simulink model "exercise02_simulation_model_solution_partA_R2025b"  (R2025b)
settings: Solver=VariableStepAuto  StartTime=0.0  StopTime=10.0  RelTol=1e-3
PreLoadFcn:
  | exercise02_simulation_parameters
undefined symbols (not defined in the file or in its folder): g, g_vec, K_lqr_full_state, nrotor_initial_condition, nrotor_initial_conditions, nrotor_vehicle, reference, sigbuilder_block
libraries: vrlib x1
settings Model: Creator=resjoehr  LastModifiedBy=diego
settings DataIOCC: SaveFormat=Array  StreamToWks=off  ReturnWorkspaceOutputs=off

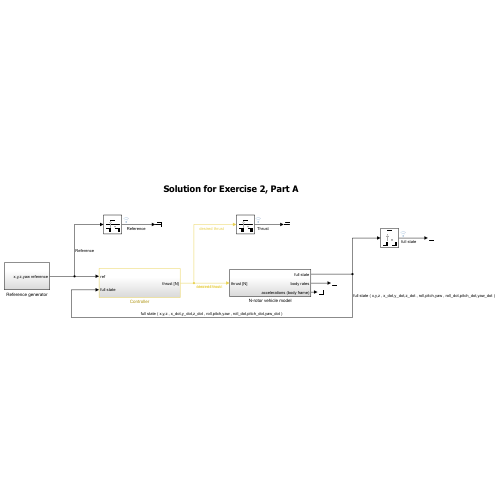
[thumbnail: Simulink's stored preview of the top-level diagram]
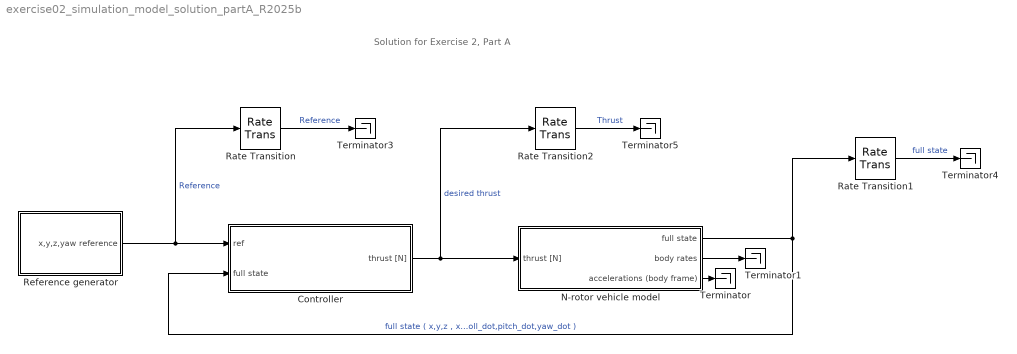
== system exercise02_simulation_model_solution_partA_R2025b ==
  note: Solution for Exercise 2, Part A
  Controller : Subsystem
  N-rotor vehicle model : Subsystem
  Rate Transition : RateTransition  OutPortSampleTime=0.05
  Rate Transition1 : RateTransition  OutPortSampleTime=0.05
  Rate Transition2 : RateTransition  OutPortSampleTime=0.05
  Reference generator : Subsystem
  Terminator{,1,3..5} (5 alike) : Terminator
  wires:
  N-rotor vehicle model/2(body rates) -> Terminator1/1
  Reference generator/1(x,y,z,yaw reference) -> Rate Transition/1, Controller/1(ref)  "Reference"
  N-rotor vehicle model/3(accelerations (body frame)) -> Terminator/1
  N-rotor vehicle model/1(full state) -> Controller/2(full state), Rate Transition1/1  "full state ( x,y,z , x_dot,y_dot,z_dot , roll,pitch,yaw , roll_dot,pitch_dot,yaw_dot )"
  Controller/1(thrust [N]) -> Rate Transition2/1, N-rotor vehicle model/1(thrust [N])  "desired thrust"
  Rate Transition1/1 -> Terminator4/1  "full state"
  Rate Transition/1 -> Terminator3/1  "Reference"
  Rate Transition2/1 -> Terminator5/1  "Thrust"

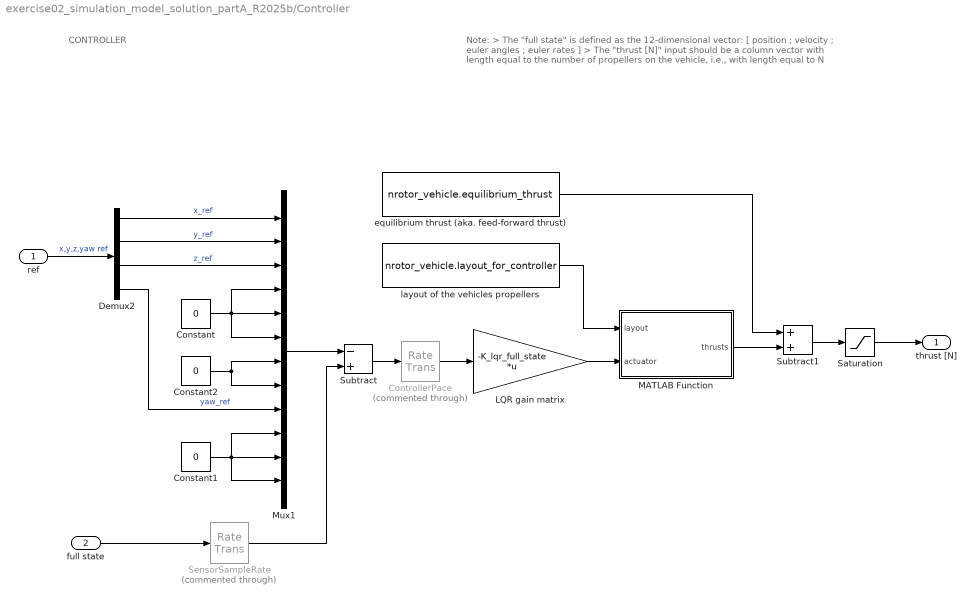
== system exercise02_simulation_model_solution_partA_R2025b/Controller ==
  note: CONTROLLER
  note: Note:
      | > The "full state" is defined as the 12-dimensional vector:
      | [ position ; velocity ; euler angles ; euler rates ]
      | > The "thrust [N]" input should be a column vector with
      | length equal to the number of propellers on the vehicle,
      | i.e., with length equal to N
  ref : Inport
  full state : Inport  Port=2
  Constant : Constant  Value=0
  Constant1 : Constant  Value=0
  Constant2 : Constant  Value=0
  ControllerPace : RateTransition  Commented=through  OutPortSampleTime=0.005
  Demux2 : Demux
  LQR gain matrix : Gain  Gain=-K_lqr_full_state  Multiplication=Matrix(K*u)
  MATLAB Function : MATLAB Function  TreatAsAtomicUnit=on
  Mux1 : Mux  Inputs=12
  Saturation : Saturate  UpperLimit=nrotor_vehicle.thrust_max  LowerLimit=nrotor_vehicle.thrust_min  ZeroCross=off
  SensorSampleRate : RateTransition  Commented=through  OutPortSampleTime=0.005
  Subtract : Sum  Inputs=-+
  Subtract1 : Sum
  equilibrium thrust (aka. feed-forward thrust) : Constant  Value=nrotor_vehicle.equilibrium_thrust
  layout of the vehicles propellers : Constant  Value=nrotor_vehicle.layout_for_controller
  thrust [N] : Outport  VectorParamsAs1DForOutWhenUnconnected=off
  wires:
  Saturation/1 -> thrust [N]/1
  ref/1 -> Demux2/1  "x,y,z,yaw ref"
  Mux1/1 -> Subtract/1
  Demux2/1 -> Mux1/1  "x_ref"
  Demux2/2 -> Mux1/2  "y_ref"
  Demux2/3 -> Mux1/3  "z_ref"
  Constant/1 -> Mux1/6, Mux1/5, Mux1/4
  full state/1 -> SensorSampleRate/1
  Subtract/1 -> ControllerPace/1
  LQR gain matrix/1 -> MATLAB Function/2(actuator)
  Subtract1/1 -> Saturation/1
  equilibrium thrust (aka. feed-forward thrust)/1 -> Subtract1/1
  Constant1/1 -> Mux1/11, Mux1/12, Mux1/10
  Constant2/1 -> Mux1/8, Mux1/7
  Demux2/4 -> Mux1/9  "yaw_ref"
  MATLAB Function/1(thrusts) -> Subtract1/2
  layout of the vehicles propellers/1 -> MATLAB Function/1(layout)
  SensorSampleRate/1 -> Subtract/2
  ControllerPace/1 -> LQR gain matrix/1

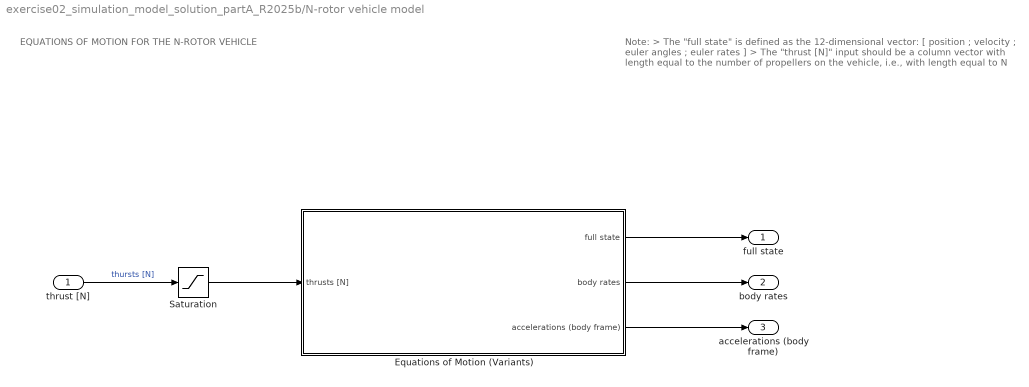
== system exercise02_simulation_model_solution_partA_R2025b/N-rotor vehicle model ==
  note: Note:
      | > The "full state" is defined as the 12-dimensional vector:
      | [ position ; velocity ; euler angles ; euler rates ]
      | > The "thrust [N]" input should be a column vector with
      | length equal to the number of propellers on the vehicle,
      | i.e., with length equal to N
  note: EQUATIONS OF MOTION FOR THE N-ROTOR VEHICLE
  thrust [N] : Inport
  Equations of Motion (Variants) : Subsystem  Variant=on  VariantControlMode=label  LabelModeActiveChoice=Choice_2
  Saturation : Saturate  UpperLimit=nrotor_vehicle.thrust_max  LowerLimit=nrotor_vehicle.thrust_min
  full state : Outport  VectorParamsAs1DForOutWhenUnconnected=off
  body rates : Outport  Port=2  VectorParamsAs1DForOutWhenUnconnected=off
  accelerations (body frame) : Outport  Port=3  VectorParamsAs1DForOutWhenUnconnected=off
  wires:
  thrust [N]/1 -> Saturation/1  "thursts [N]"
  Saturation/1 -> Equations of Motion (Variants)/1(thrusts [N])
  Equations of Motion (Variants)/2(body rates) -> body rates/1
  Equations of Motion (Variants)/1(full state) -> full state/1
  Equations of Motion (Variants)/3(accelerations (body frame)) -> accelerations (body frame)/1

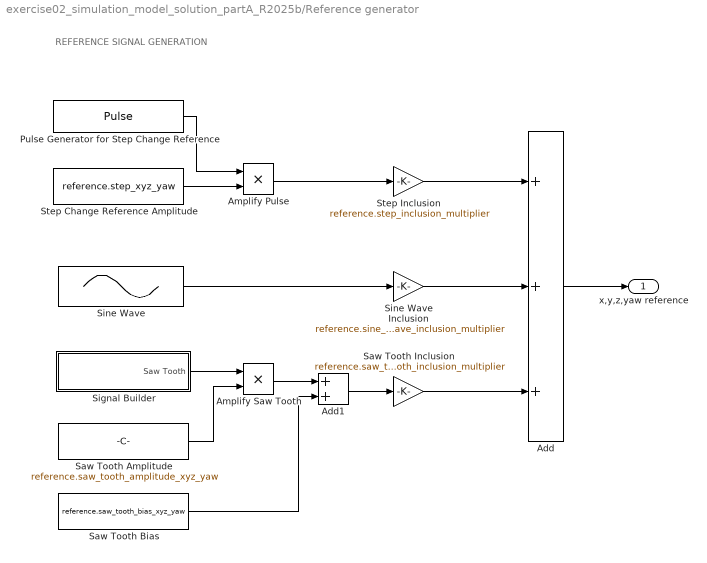
== system exercise02_simulation_model_solution_partA_R2025b/Reference generator ==
  note: REFERENCE SIGNAL GENERATION
  Add : Sum  Inputs=+++
  Add1 : Sum
  Amplify Pulse : Product
  Amplify Saw Tooth : Product
  Pulse Generator for Step Change Reference : DiscretePulseGenerator  PulseType=Time based  Period=reference.step_period*2  PulseWidth=50
  Saw Tooth Amplitude : Constant  Value=reference.saw_tooth_amplitude_xyz_yaw
  Saw Tooth Bias : Constant  Value=reference.saw_tooth_bias_xyz_yaw
  Saw Tooth Inclusion : Gain  Gain=reference.saw_tooth_inclusion_multiplier
  Signal Builder : Subsystem  Tag=STV Subsys  LoadFcn=sigbuilder_block('load');  StartFcn=sigbuilder_block('start');  StopFcn=sigbuilder_block('stop');  ClipboardFcn=sigbuilder_block('clipboard');  mask(Sigbuilder block){tuvar=[0:10]}
      mask help: Simulink:masks:SigbuilderBlock_MD
      mask init:
      | if ~strcmp(get_param(bdroot(gcbh),'SimulationStatus'),'stopped') tuvar = sigbuilder_block('maskInit'); end
      settings: CopyFcn=sigbuilder_block('copy');  DeleteFcn=sigbuilder_block('delete');  ModelCloseFcn=sigbuilder_block('modelClose');  PreSaveFcn=sigbuilder_block('preSave');  PauseFcn=sigbuilder_block('pause');  ContinueFcn=sigbuilder_block('continue');  NameChangeFcn=sigbuilder_block('namechange');  OpenFcn=sigbuilder_block('open',[1782.75 377.25 895.5 539.25 ]);  CloseFcn=sigbuilder_block('close');
      mask Display: plot(0, 0, 100, 100,[2, 2, 32, 32, 2], [68, 8, 8, 68, 68],[32, 2], [38, 38], [32, 19, 2],[53, 60, 44], [32, 17, 17, 2],[16, 16, 31, 31]);txt = getActiveGroup(gcbh);text(2, 100, txt,'verticalAlignment', 'top');
  Sine Wave : Sin  Amplitude=reference.sine_amplitude_xyz_yaw  Bias=reference.sine_bias_xyz_yaw  Frequency=2*pi()/reference.sine_period  SampleTime=0
  Sine Wave Inclusion : Gain  Gain=reference.sine_wave_inclusion_multiplier
  Step Change Reference Amplitude : Constant  Value=reference.step_xyz_yaw
  Step Inclusion : Gain  Gain=reference.step_inclusion_multiplier
  x,y,z,yaw reference : Outport  VectorParamsAs1DForOutWhenUnconnected=off
  wires:
  Step Change Reference Amplitude/1 -> Amplify Pulse/2
  Pulse Generator for Step Change Reference/1 -> Amplify Pulse/1
  Sine Wave/1 -> Sine Wave Inclusion/1
  Add/1 -> x,y,z,yaw reference/1
  Step Inclusion/1 -> Add/1
  Sine Wave Inclusion/1 -> Add/2
  Amplify Pulse/1 -> Step Inclusion/1
  Saw Tooth Inclusion/1 -> Add/3
  Signal Builder/1(Saw Tooth) -> Amplify Saw Tooth/1
  Saw Tooth Amplitude/1 -> Amplify Saw Tooth/2
  Amplify Saw Tooth/1 -> Add1/1
  Add1/1 -> Saw Tooth Inclusion/1
  Saw Tooth Bias/1 -> Add1/2

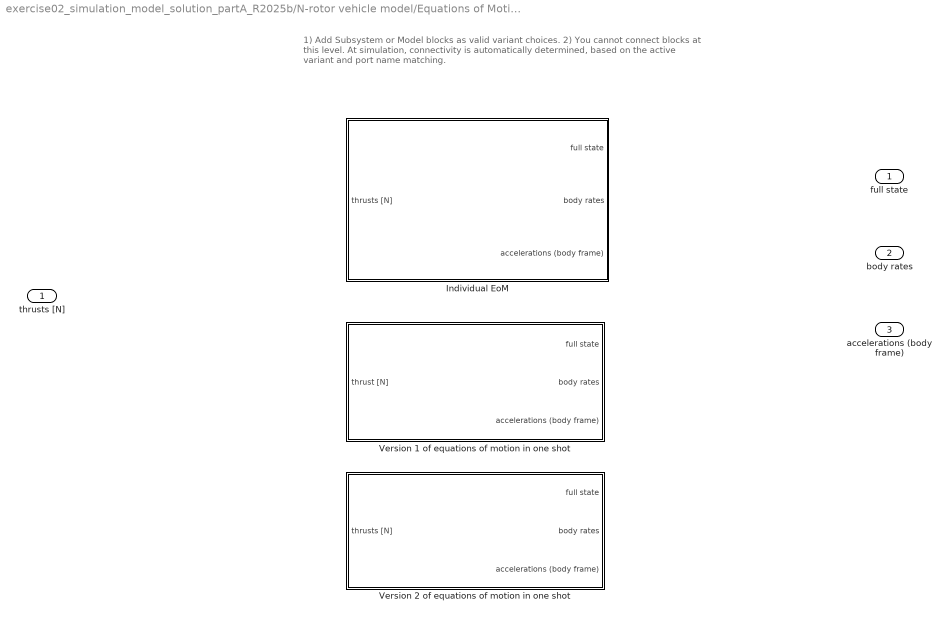
== system exercise02_simulation_model_solution_partA_R2025b/N-rotor vehicle model/Equations of Motion (Variants) ==
  note: 1) Add Subsystem or Model blocks as valid variant choices.
      | 2) You cannot connect blocks at this level. At simulation, connectivity is automatically
      | determined, based on the active variant and port name matching.
  thrusts [N] : Inport
  Individual EoM : Subsystem  VariantControl=Choice
  Version 1 of equations of motion in one shot : Subsystem  VariantControl=Choice_1
  Version 2 of equations of motion in one shot : Subsystem  VariantControl=Choice_2
  full state : Outport
  body rates : Outport  Port=2
  accelerations (body frame) : Outport  Port=3

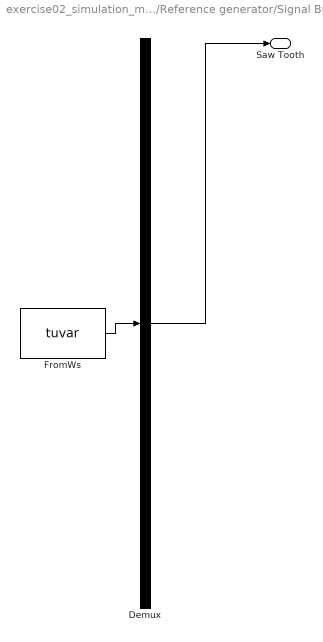
== system exercise02_simulation_model_solution_partA_R2025b/Reference generator/Signal Builder ==
  Demux : Demux  Tag=STV Demux  Outputs=1
      settings: DisplayOption=none
  FromWs : FromWorkspace  Tag=STV FromWs  VariableName=tuvar
      SigBuilderData=|
      | common.afterFinalStr = 'Extrapolate'
      | common.sampleTime = 0
      | dataSet.timeRange = [0 10]
      | dataSet.name = 'Group 1'
      | sbobj.Groups.Name = 'Group 1'
      | sbobj.Groups.Signals.Name = 'Saw Tooth'
      | sbobj.Groups.Signals.XData = [0 2.5 7.5 10]
      | sbobj.Groups.Signals.YData = [0 1.01 -1 0]
  Saw Tooth : Outport  Tag=STV Outport  VectorParamsAs1DForOutWhenUnconnected=off
  wires:
  Demux/1 -> Saw Tooth/1
  FromWs/1 -> Demux/1

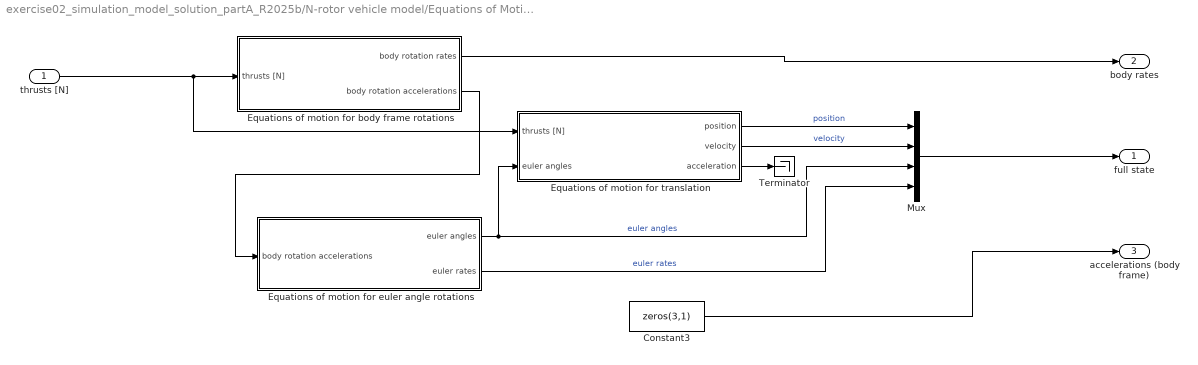
== system exercise02_simulation_model_solution_partA_R2025b/N-rotor vehicle model/Equations of Motion (Variants)/Individual EoM ==
  thrusts [N] : Inport
  Constant3 : Constant  Value=zeros(3,1)
  Equations of motion for body frame rotations : Subsystem
  Equations of motion for euler angle rotations : Subsystem
  Equations of motion for translation : Subsystem
  Mux : Mux
  Terminator : Terminator
  full state : Outport
  body rates : Outport  Port=2
  accelerations (body frame) : Outport  Port=3
  wires:
  Equations of motion for euler angle rotations/1(euler angles) -> Equations of motion for translation/2(euler angles), Mux/3  "euler angles"
  Equations of motion for body frame rotations/2("body rotation accelerations ") -> Equations of motion for euler angle rotations/1(body rotation accelerations)
  Equations of motion for translation/1(position) -> Mux/1  "position"
  thrusts [N]/1 -> Equations of motion for translation/1(thrusts [N]), Equations of motion for body frame rotations/1(thrusts [N])
  Equations of motion for body frame rotations/1(body rotation rates) -> body rates/1
  Equations of motion for euler angle rotations/2(euler rates) -> Mux/4  "euler rates"
  Equations of motion for translation/3(acceleration) -> Terminator/1
  Equations of motion for translation/2(velocity) -> Mux/2  "velocity"
  Mux/1 -> full state/1
  Constant3/1 -> accelerations (body frame)/1

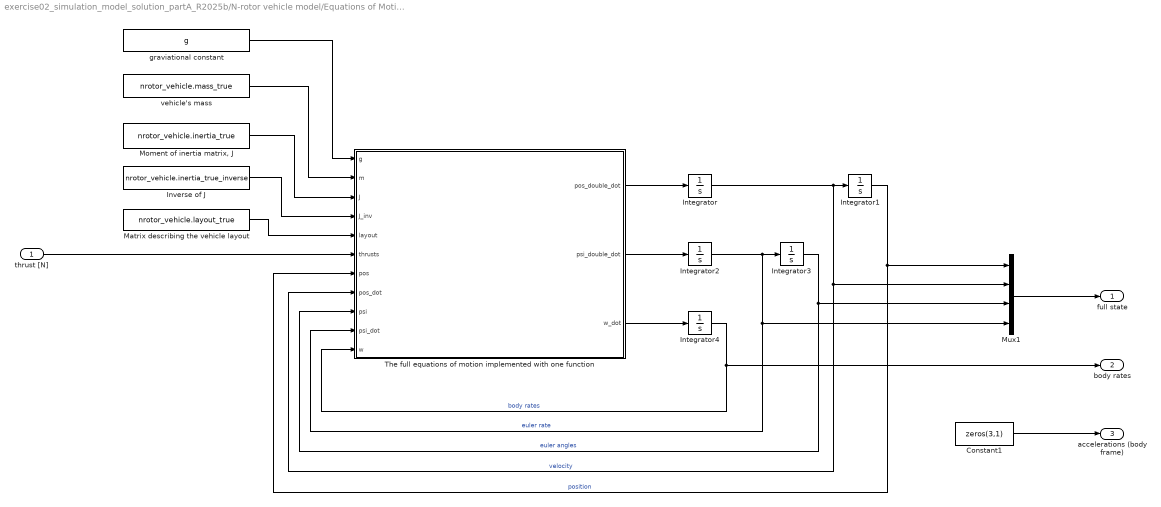
== system exercise02_simulation_model_solution_partA_R2025b/N-rotor vehicle model/Equations of Motion (Variants)/Version 1 of equations of motion in one shot ==
  thrust [N] : Inport
  Constant1 : Constant  Value=zeros(3,1)
  Integrator : Integrator  InitialCondition=nrotor_initial_condition.p_dot
  Integrator1 : Integrator  InitialCondition=nrotor_initial_condition.p
  Integrator2 : Integrator  InitialCondition=nrotor_initial_condition.psi_dot
  Integrator3 : Integrator  InitialCondition=nrotor_initial_condition.psi
  Integrator4 : Integrator  InitialCondition=nrotor_initial_condition.body_rates
  Inverse of J : Constant  Value=nrotor_vehicle.inertia_true_inverse
  Matrix describing the vehicle layout : Constant  Value=nrotor_vehicle.layout_true
  "Moment of inertia matrix, J" : Constant  Value=nrotor_vehicle.inertia_true
  Mux1 : Mux
  The full equations of motion implemented with one function : MATLAB Function  TreatAsAtomicUnit=on
  graviational constant : Constant  Value=g
  vehicle's mass : Constant  Value=nrotor_vehicle.mass_true
  full state : Outport  VectorParamsAs1DForOutWhenUnconnected=off
  body rates : Outport  Port=2  VectorParamsAs1DForOutWhenUnconnected=off
  accelerations (body frame) : Outport  Port=3  VectorParamsAs1DForOutWhenUnconnected=off
  wires:
  Integrator2/1 -> Integrator3/1, Mux1/4, The full equations of motion implemented with one function/10(psi_dot)  "euler rate"
  The full equations of motion implemented with one function/2(psi_double_dot) -> Integrator2/1
  vehicle's mass/1 -> The full equations of motion implemented with one function/2(m)
  Matrix describing the vehicle layout/1 -> The full equations of motion implemented with one function/5(layout)
  The full equations of motion implemented with one function/3(w_dot) -> Integrator4/1
  Integrator1/1 -> The full equations of motion implemented with one function/7(pos), Mux1/1  "position"
  Integrator/1 -> The full equations of motion implemented with one function/8(pos_dot), Mux1/2, Integrator1/1  "velocity"
  Constant1/1 -> accelerations (body frame)/1
  The full equations of motion implemented with one function/1(pos_double_dot) -> Integrator/1
  thrust [N]/1 -> The full equations of motion implemented with one function/6(thrusts)
  "Moment of inertia matrix, J"/1 -> The full equations of motion implemented with one function/3(J)
  Inverse of J/1 -> The full equations of motion implemented with one function/4(J_inv)
  Integrator3/1 -> The full equations of motion implemented with one function/9(psi), Mux1/3  "euler angles"
  Integrator4/1 -> body rates/1, The full equations of motion implemented with one function/11(w)  "body rates"
  Mux1/1 -> full state/1
  graviational constant/1 -> The full equations of motion implemented with one function/1(g)

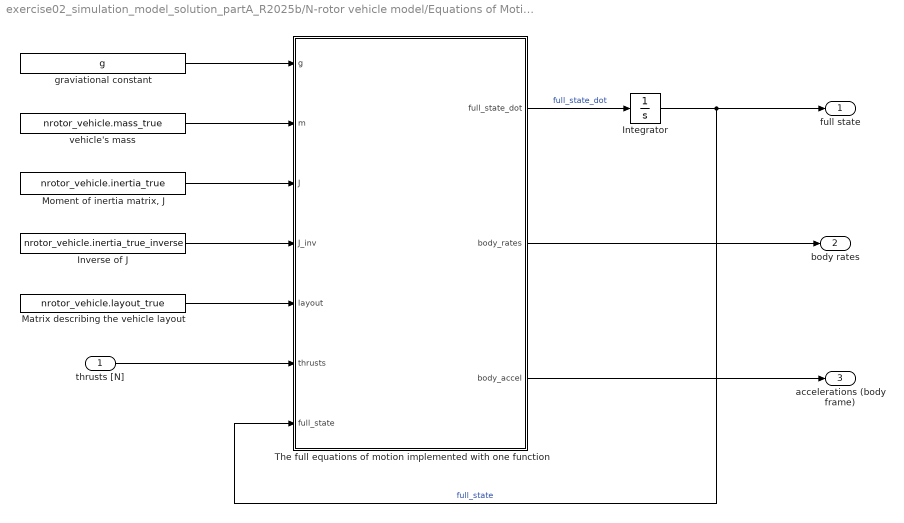
== system exercise02_simulation_model_solution_partA_R2025b/N-rotor vehicle model/Equations of Motion (Variants)/Version 2 of equations of motion in one shot ==
  thrusts [N] : Inport
  Integrator : Integrator  InitialCondition=nrotor_initial_conditions
  Inverse of J : Constant  Value=nrotor_vehicle.inertia_true_inverse
  Matrix describing the vehicle layout : Constant  Value=nrotor_vehicle.layout_true
  "Moment of inertia matrix, J" : Constant  Value=nrotor_vehicle.inertia_true
  The full equations of motion implemented with one function : MATLAB Function  TreatAsAtomicUnit=on
  graviational constant : Constant  Value=g
  vehicle's mass : Constant  Value=nrotor_vehicle.mass_true
  full state : Outport  VectorParamsAs1DForOutWhenUnconnected=off
  body rates : Outport  Port=2  VectorParamsAs1DForOutWhenUnconnected=off
  accelerations (body frame) : Outport  Port=3  VectorParamsAs1DForOutWhenUnconnected=off
  wires:
  thrusts [N]/1 -> The full equations of motion implemented with one function/6(thrusts)
  The full equations of motion implemented with one function/2(body_rates) -> body rates/1
  Inverse of J/1 -> The full equations of motion implemented with one function/4(J_inv)
  "Moment of inertia matrix, J"/1 -> The full equations of motion implemented with one function/3(J)
  graviational constant/1 -> The full equations of motion implemented with one function/1(g)
  vehicle's mass/1 -> The full equations of motion implemented with one function/2(m)
  Matrix describing the vehicle layout/1 -> The full equations of motion implemented with one function/5(layout)
  Integrator/1 -> The full equations of motion implemented with one function/7(full_state), full state/1  "full_state"
  The full equations of motion implemented with one function/1(full_state_dot) -> Integrator/1  "full_state_dot"
  The full equations of motion implemented with one function/3(body_accel) -> accelerations (body frame)/1

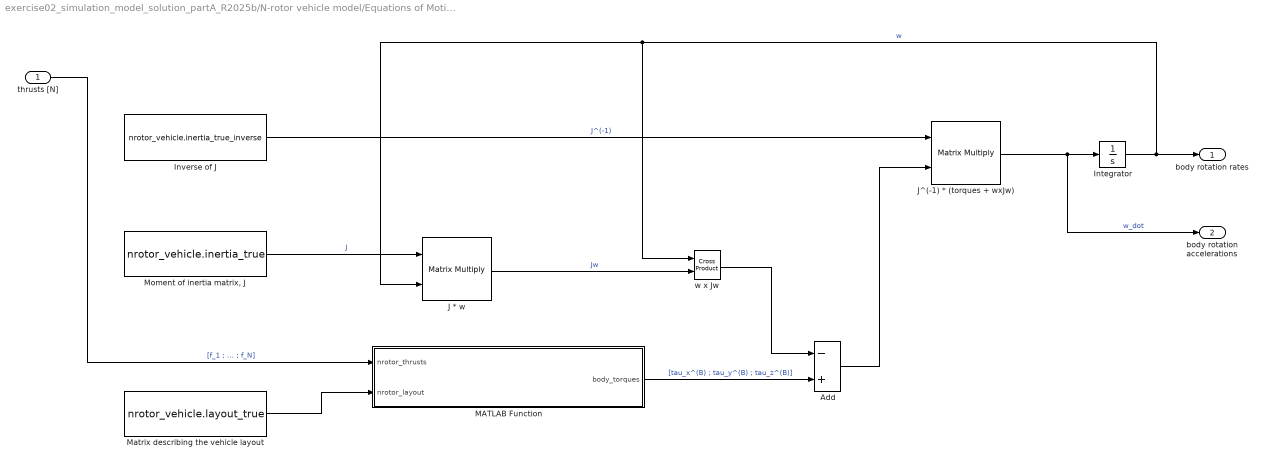
== system exercise02_simulation_model_solution_partA_R2025b/N-rotor vehicle model/Equations of Motion (Variants)/Individual EoM/Equations of motion for body frame rotations ==
  thrusts [N] : Inport
  Add : Sum  Inputs=-+
  Integrator : Integrator  InitialCondition=nrotor_initial_condition.body_rates
  Inverse of J : Constant  Value=nrotor_vehicle.inertia_true_inverse
  J * w : Product  Multiplication=Matrix(*)  RndMeth=Zero
  J^(-1) * (torques + wxJw) : Product  Multiplication=Matrix(*)  RndMeth=Zero
  MATLAB Function : MATLAB Function  TreatAsAtomicUnit=on
  Matrix describing the vehicle layout : Constant  Value=nrotor_vehicle.layout_true
  "Moment of inertia matrix, J" : Constant  Value=nrotor_vehicle.inertia_true
  w x Jw : vrlib/Utilities/Cross Product
  body rotation rates : Outport  VectorParamsAs1DForOutWhenUnconnected=off
  "body rotation accelerations " : Outport  Port=2  VectorParamsAs1DForOutWhenUnconnected=off
  wires:
  Integrator/1 -> J * w/2, w x Jw/1, body rotation rates/1  "w"
  Add/1 -> J^(-1) * (torques + wxJw)/2
  w x Jw/1 -> Add/1
  J * w/1 -> w x Jw/2  "Jw"
  MATLAB Function/1(body_torques) -> Add/2  "[tau_x^(B) ; tau_y^(B) ; tau_z^(B)]"
  Inverse of J/1 -> J^(-1) * (torques + wxJw)/1  "J^(-1)"
  thrusts [N]/1 -> MATLAB Function/1(nrotor_thrusts)  "[f_1 ; ... ; f_N]"
  "Moment of inertia matrix, J"/1 -> J * w/1  "J"
  J^(-1) * (torques + wxJw)/1 -> "body rotation accelerations "/1, Integrator/1  "w_dot"
  Matrix describing the vehicle layout/1 -> MATLAB Function/2(nrotor_layout)

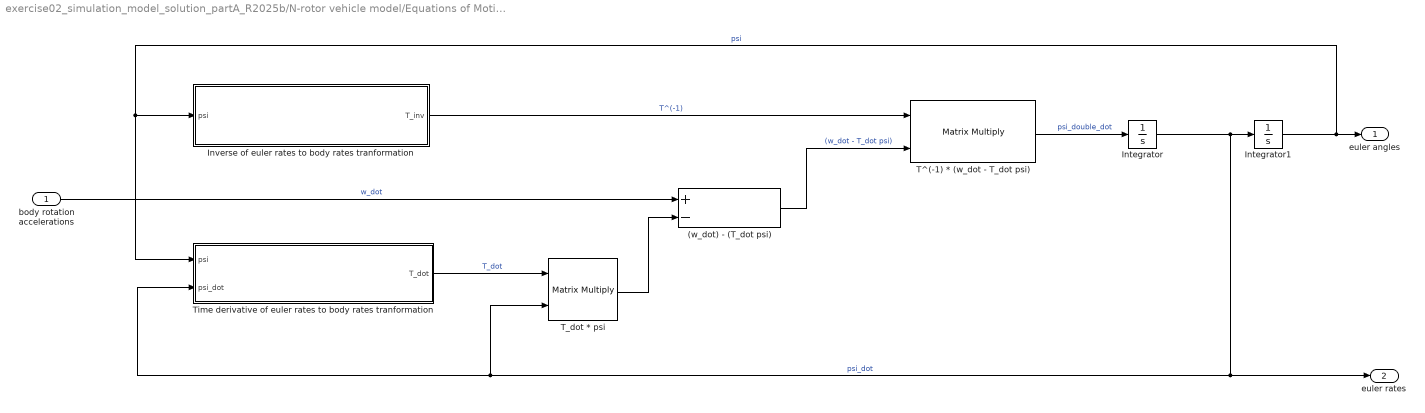
== system exercise02_simulation_model_solution_partA_R2025b/N-rotor vehicle model/Equations of Motion (Variants)/Individual EoM/Equations of motion for euler angle rotations ==
  body rotation accelerations : Inport
  (w_dot) - (T_dot psi) : Sum  Inputs=+-
  Integrator : Integrator  InitialCondition=nrotor_initial_condition.psi_dot
  Integrator1 : Integrator  InitialCondition=nrotor_initial_condition.psi
  Inverse of euler rates to body rates tranformation : MATLAB Function  TreatAsAtomicUnit=on
  T^(-1) * (w_dot - T_dot psi) : Product  Multiplication=Matrix(*)  RndMeth=Zero
  T_dot * psi : Product  Multiplication=Matrix(*)  RndMeth=Zero
  Time derivative of euler rates to body rates tranformation : MATLAB Function  TreatAsAtomicUnit=on
  euler angles : Outport  VectorParamsAs1DForOutWhenUnconnected=off
  euler rates : Outport  Port=2  VectorParamsAs1DForOutWhenUnconnected=off
  wires:
  T^(-1) * (w_dot - T_dot psi)/1 -> Integrator/1  "psi_double_dot"
  Time derivative of euler rates to body rates tranformation/1(T_dot) -> T_dot * psi/1  "T_dot"
  Inverse of euler rates to body rates tranformation/1(T_inv) -> T^(-1) * (w_dot - T_dot psi)/1  "T^(-1)"
  T_dot * psi/1 -> (w_dot) - (T_dot psi)/2
  (w_dot) - (T_dot psi)/1 -> T^(-1) * (w_dot - T_dot psi)/2  "(w_dot - T_dot psi)"
  Integrator1/1 -> Time derivative of euler rates to body rates tranformation/1(psi), Inverse of euler rates to body rates tranformation/1(psi), euler angles/1  "psi"
  body rotation accelerations/1 -> (w_dot) - (T_dot psi)/1  "w_dot"
  Integrator/1 -> Integrator1/1, T_dot * psi/2, Time derivative of euler rates to body rates tranformation/2(psi_dot), euler rates/1  "psi_dot"

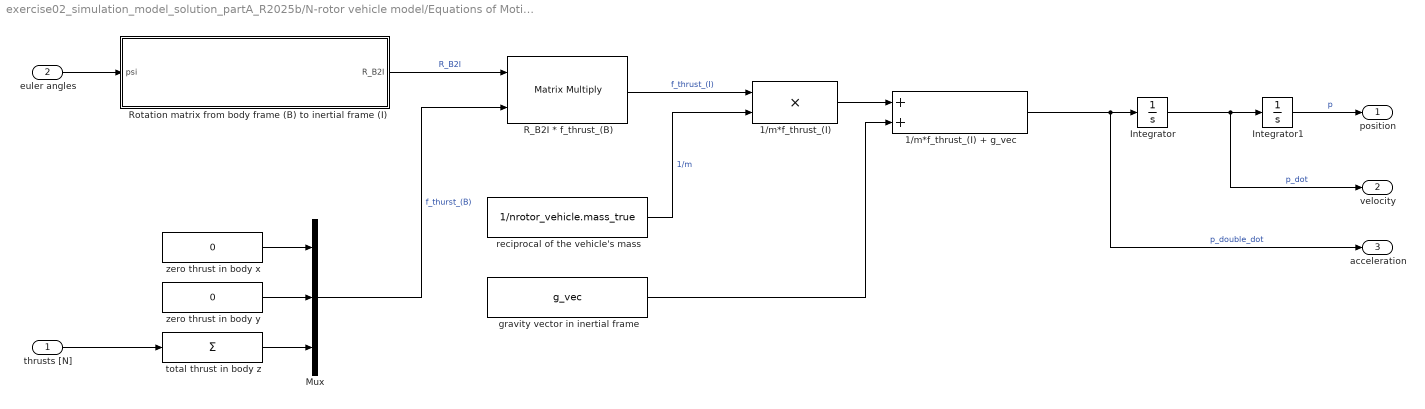
== system exercise02_simulation_model_solution_partA_R2025b/N-rotor vehicle model/Equations of Motion (Variants)/Individual EoM/Equations of motion for translation ==
  thrusts [N] : Inport
  euler angles : Inport  Port=2
  1/m*f_thrust_(I) : Product
  1/m*f_thrust_(I) + g_vec : Sum
  Integrator : Integrator  InitialCondition=nrotor_initial_condition.p_dot
  Integrator1 : Integrator  InitialCondition=nrotor_initial_condition.p
  Mux : Mux  Inputs=3
  R_B2I * f_thrust_(B) : Product  Multiplication=Matrix(*)  RndMeth=Zero
  Rotation matrix from body frame (B) to inertial frame (I) : MATLAB Function  TreatAsAtomicUnit=on
  gravity vector in inertial frame : Constant  Value=g_vec
  reciprocal of the vehicle's mass : Constant  Value=1/nrotor_vehicle.mass_true
  total thrust in body z : Sum  Inputs=+
  zero thrust in body x : Constant  Value=0
  zero thrust in body y : Constant  Value=0
  position : Outport  VectorParamsAs1DForOutWhenUnconnected=off
  velocity : Outport  Port=2  VectorParamsAs1DForOutWhenUnconnected=off
  acceleration : Outport  Port=3  VectorParamsAs1DForOutWhenUnconnected=off
  wires:
  gravity vector in inertial frame/1 -> 1/m*f_thrust_(I) + g_vec/2
  euler angles/1 -> Rotation matrix from body frame (B) to inertial frame (I)/1(psi)
  Rotation matrix from body frame (B) to inertial frame (I)/1(R_B2I) -> R_B2I * f_thrust_(B)/1  "R_B2I"
  1/m*f_thrust_(I) + g_vec/1 -> acceleration/1, Integrator/1  "p_double_dot"
  Integrator/1 -> Integrator1/1, velocity/1  "p_dot"
  R_B2I * f_thrust_(B)/1 -> 1/m*f_thrust_(I)/1  "f_thrust_(I)"
  Integrator1/1 -> position/1  "p"
  thrusts [N]/1 -> total thrust in body z/1
  total thrust in body z/1 -> Mux/3
  zero thrust in body y/1 -> Mux/2
  zero thrust in body x/1 -> Mux/1
  Mux/1 -> R_B2I * f_thrust_(B)/2  "f_thurst_(B)"
  reciprocal of the vehicle's mass/1 -> 1/m*f_thrust_(I)/2  "1/m"
  1/m*f_thrust_(I)/1 -> 1/m*f_thrust_(I) + g_vec/1

== matlab function exercise02_simulation_model_solution_partA_R2025b/N-rotor vehicle model/Equations of Motion (Variants)/Individual EoM/Equations of motion for euler angle rotations/Inverse of euler rates to body rates tranformation ==
  data: psi input; T_inv output size=[3,3]
function T_inv = compute_T_inverse(psi)
% ----------------------------------------------------------------------- %
% DESCRIPTION:
% This function computes the inverse of the euler rates to body rates
% transformation matrix for a given set of intrinsic (roll,pitch,yaw) euler
% angles.
%
%
% INPUT ARGUMENTS:
% psi [radians]
% > This is a vector of length 3, and each element represents the roll,
%   pitch, and yaw intrinsic euler angles respectively, in units of radians
%
%
% RETURN ARGUMENTS:
% T_inv
% > This is a 3-by-3 matrix this is the inverse of the euler rates to body
%   rates transformation matrix
%
%
% DATA FORMAT ASSUMPTIONS:
% > That the "psi" is ordered as:
%   psi = [ roll ; pitch ; yaw ];
%
% ----------------------------------------------------------------------- %

% Extract each euler angles
r  =  psi(1);  % Roll
p  =  psi(2);  % Pitch
%y  =  psi(3); % Yaw, which is not need in this function

% Compute the T inverse matrix:
T_inv = [...
        1  ,  sin(r)*tan(p)  ,   cos(r)*tan(p)  ;...
        0  ,  cos(r)         ,  -sin(r)         ;...
        0  ,  sin(r)*sec(p)  ,   cos(r)*sec(p)   ...
    ];
 
end

== matlab function exercise02_simulation_model_solution_partA_R2025b/N-rotor vehicle model/Equations of Motion (Variants)/Individual EoM/Equations of motion for body frame rotations/MATLAB Function ==
  data: nrotor_thrusts input; body_torques output; nrotor_layout input
function body_torques = convert_thrusts_to_torques(nrotor_thrusts,nrotor_layout)
% ----------------------------------------------------------------------- %
% DESCRIPTION:
% This function converts the thrust produced from each rotor to the torques
% about the body frame axes
%
%
% INPUT ARGUMENTS:
% nrotor_thrusts
% > This is a colulmn vector with length equal to the number of propellers
%   on the N-rotor vehicle, and each element represents the thrust force in
%   Newtons being produced by the respective propeller
%
% nrotor_layout
% > This is a matrix that specifies the layout via the following format:
% nrotor_vehicle_layout = [...
%       x_1  ,  x_2  ,  ...  ,  x_{N-1}  ,  x_{N}  ;...
%       y_1  ,  y_2  ,  ...  ,  y_{N-1}  ,  y_{N}  ;...
%       c_1  ,  c_2  ,  ...  ,  c_{N-1}  ,  c_{N}   ...
%   ];
% where:
%   > x_i   is the x coordinate of propeller "i" relative to the CoG
%   > y_i   is the y coordinate of propeller "i" relative to the CoG
%   > c_i   is the thurst to torque coefficient of the propeller, with the
%           sign used to indicate the propeller's direction of rotation,
%           +ve indicates clock-wise propeller rotation.
%
%
% RETURN ARGUMENTS:
% body_torques
% > This is a column vector of length 3 which contains the torque about the
% body frame axes x,y,z respectively
%
%
% DATA FORMAT ASSUMPTIONS:
% > That the "nrotor_thrusts" input argument is a column vector
% > That the number of columns of "nrotor_layout" equals the length of
%   "nrotor_thrusts"
%
% ----------------------------------------------------------------------- %


body_torques = [...
        nrotor_layout(2,:) ;...
       -nrotor_layout(1,:) ;...
        nrotor_layout(3,:)  ...
    ]...
    * nrotor_thrusts;

== matlab function exercise02_simulation_model_solution_partA_R2025b/N-rotor vehicle model/Equations of Motion (Variants)/Individual EoM/Equations of motion for euler angle rotations/Time derivative of euler rates to body rates tranformation ==
  data: psi input; T_dot output size=[3,3]; psi_dot input
function T_dot = compute_T_dot(psi,psi_dot)
% ----------------------------------------------------------------------- %
% DESCRIPTION:
% This function computes the time derivative of the euler rates to body
% rates transformation matrix for a given set of intrinsic (roll,pitch,yaw)
% euler angles and their angular velocities (roll_dot,pitch_dot,yaw_dot).
%
%
% INPUT ARGUMENTS:
% psi [radians]
% > This is a vector of length 3, and each element represents the roll,
%   pitch, and yaw intrinsic euler angles respectively, in units of radians
%
% psi_dot [radians/second]
% > This is a vector of length 3, and each element represents the angular
%   velocity of the roll, pitch, and yaw intrinsic euler angles
%   respectively, in units of radians per second
%
%
% RETURN ARGUMENTS:
% T_dot
% > This is a 3-by-3 matrix this is the time derivative of the euler rates
%   to body rates transformation matrix
%
%
% DATA FORMAT ASSUMPTIONS:
% > That the "psi" is ordered as:
%   psi = [ roll ; pitch ; yaw ];
% > And equivalently that the "psi_dot" is ordered as:
%   psi_dot = [ roll_dot ; pitch_dot ; yaw_dot ];
%
% ----------------------------------------------------------------------- %

% Extract each euler angles
%r  =  psi(1);  % Roll
%p  =  psi(2);  % Pitch
%y  =  psi(3); % Yaw, which is not need in this function

r  =  psi(1);  % Roll
p  =  psi(2);  % Pitch
%y  =  psi(3); % Yaw, which is not need in this function

rdot  =  psi_dot(1);  % Roll  angular velocity
pdot  =  psi_dot(2);  % Pitch angular velocity
%ydot  =  psi_dot(3); % Yaw   angular velocity, also not needed

% Compute the time derivative of the T matrix:
T_dot = [...
        0  ,   0            ,  -pdot*cos(p)                            ;...
        0  ,  -rdot*sin(r)  ,   rdot*cos(r)*cos(p)-pdot*sin(r)*sin(p)  ;...
        0  ,  -rdot*cos(r)  ,  -rdot*sin(r)*cos(p)-pdot*cos(r)*sin(p)   ...
    ];

end

== matlab function exercise02_simulation_model_solution_partA_R2025b/N-rotor vehicle model/Equations of Motion (Variants)/Individual EoM/Equations of motion for translation/Rotation matrix from body frame (B) to inertial frame (I) ==
  data: psi input; R_B2I output size=[3,3]
function R_B2I = compute_rotation_matrix_body2inertial(psi)
% ----------------------------------------------------------------------- %
% DESCRIPTION:
% This function computes the rottaion matrix from the body frame (B) to the
% inertial frame (I) for a given set of intrinsic (roll,pitch,yaw) euler
% angles.
%
%
% INPUT ARGUMENTS:
% psi [radians]
% > This is a vector of length 3, and each element represents the roll,
%   pitch, and yaw intrinsic euler angles respectively, in units of radians
%
%
% RETURN ARGUMENTS:
% R_B2I
% > This is a 3-by-3 matrix this is the rotation matrix that converts a
%   vector in the body frame coordiantes to its equivalent in the inertial
%   frame coordinates
%
%
% DATA FORMAT ASSUMPTIONS:
% > That the "psi" is ordered as:
%   psi = [ roll ; pitch ; yaw ];
%
% ----------------------------------------------------------------------- %


% Extract each euler angles
r  =  psi(1);  % Roll
p  =  psi(2);  % Pitch
y  =  psi(3);  % Yaw

% Compute the rotation matrix from body frame to inertial frame:
R_B2I = [...
         cos(y)*cos(p)  ,  cos(y)*sin(p)*sin(r)-sin(y)*cos(r)  ,  cos(y)*sin(p)*cos(r)+sin(y)*sin(r)  ;...
         sin(y)*cos(p)  ,  sin(y)*sin(p)*sin(r)+cos(y)*cos(r)  ,  sin(y)*sin(p)*cos(r)-cos(y)*sin(r)  ;...
        -sin(p)         ,  cos(p)*sin(r)                       ,  cos(p)*cos(r)                        ...
    ];

end

== matlab function exercise02_simulation_model_solution_partA_R2025b/Controller/MATLAB Function ==
  data: layout input; actuator input; thrusts output
function thrusts = fcn(layout,actuator)
% INPUT ARGUMENTS:
% > actuator
%   This is the desired actuator values as requested by the "u=Kx"
%   computation where "K" is the LQR controller gain matrix
% > layout
%   This describes the layout of the N-rotor vehicle, following the usual
%   convention
%
% OUTPUT ARGUMENTS
% > thrusts
%   This is the adjustment thrusts to request from each propeller of the
%   N-rotor vehicle, i.e., this should be added to the equilibrium thrusts

% STEP 1:
% Construct the "propeller-force-to-actuator" conversion matrix:
nrotor_vehicle_M = [...
        ones(1,size(layout,2)) ;...
        layout(2,:) ;...
       -layout(1,:) ;...
        layout(3,:)  ...
    ];

% STEP 2:
% Second, compute the equilibrium thrust as the solution of the
% following minimisation problem:
%     
%     minimise       sum_{i=1}^{N} thrust_i^2
%
%     subject to:    nrotor_vehicle_M * [ thrust_1 ; ... ; thrust_N ] ...
%                          == [ total_force ; body_x_torque ; body_y_torque ; body_z_torque ]
%
%     For which the solution satisfies
%     [ eye(N) , nrotor_vehicle_M' ; nrotor_vehicle_M , zeros(4,4) ] ...
%                   == [ zeros(N,1) ; actuator ]
%

% Put the number of rotors into a variable with a shorter name:
nu = size(layout,2);

% Compute the solution:
temp_solution = ...
    [ eye(nu) , nrotor_vehicle_M' ; nrotor_vehicle_M , zeros(4,4) ] ...
        \ [ zeros(nu,1) ; actuator ];

% Extract the equilibrium thrusts from the solution
thrusts = temp_solution(1:nu,1);

== matlab function exercise02_simulation_model_solution_partA_R2025b/N-rotor vehicle model/Equations of Motion (Variants)/Version 1 of equations of motion in one shot/The full equations of motion implemented with one function ==
  data: g input; m input; J input; J_inv input; layout input; thrusts input; pos_double_dot output; pos input; pos_dot input; psi input; psi_dot input; w input; psi_double_dot output; w_dot output
function [pos_double_dot,psi_double_dot,w_dot] = compute_full_equaitons_of_motion(g,m,J,J_inv,layout,thrusts,pos,pos_dot,psi,psi_dot,w)
% ----------------------------------------------------------------------- %
% DESCRIPTION:
% This function implements the full equation of motion in one function to
% simply the exposition.
%
%
% INPUT ARGUMENTS:
% m
% > This is the mass of the vehicle, in units of kilograms
%
% g
% > This is the acceleration due to gravity (typically 9.81), in units of
%   meters per second squared
%
% J
% > This is the moment of inertia matrix of the vehicle (it should be a
%   3-by3 matrix), the units of each element is kilogram meters squared
%
% J_inv
% > This is the inverse of the momement of inertia matrix, it is not
%   compute in this script to reduce the simulation run time slightly
%
% layout
% > This is a matrix that specifies the layout via the following format:
% nrotor_vehicle_layout = [...
%       x_1  ,  x_2  ,  ...  ,  x_{N-1}  ,  x_{N}  ;...
%       y_1  ,  y_2  ,  ...  ,  y_{N-1}  ,  y_{N}  ;...
%       c_1  ,  c_2  ,  ...  ,  c_{N-1}  ,  c_{N}   ...
%   ];
% where:
%   > x_i   is the x coordinate of propeller "i" relative to the CoG
%   > y_i   is the y coordinate of propeller "i" relative to the CoG
%   > c_i   is the thurst to torque coefficient of the propeller, with the
%           sign used to indicate the propeller's direction of rotation,
%           +ve indicates clock-wise propeller rotation.
%
% thrusts
% > This is a colulmn vector with length equal to the number of propellers
%   on the N-rotor vehicle, and each element represents the thrust force in
%   Newtons being produced by the respective propeller
%
% pos
% > This is a vector of length 3, and each element represent the x,y,z
%   posiiton of the body frame origin expressed in inertial frame
%   coordinates, in units of meters
% > Note, that "p" is not used in this function, but it is kept as an input
%   argument for the sake of generality
%
% pos_dot
% > This is a vector of length 3, and each element represent the x,y,z
%   linear velocity of the body frame origin expressed in inertial frame
%   coordinates, in units of meters per second
% > Note, that "p_dot" is not used in this function, but it is kept as an
%   input argument for the sake of generality
%
% psi [radians]
% > This is a vector of length 3, and each element represents the roll,
%   pitch, and yaw intrinsic euler angles respectively, in units of radians
%
% psi_dot [radians/second]
% > This is a vector of length 3, and each element represents the angular
%   velocity of the roll, pitch, and yaw intrinsic euler angles
%   respectively, in units of radians per second
%
% w
% > This is a vector of length 3, and each element represents the angular
%   velocity of the body frame as measured about the body frame's
%   coordinate axes, i.e., this is exactly what is measured by a typical
%   strap-down Inertial Measurement Unit (IMU) this is attached to the body
%   of most all flying vehicles. "w" is referred to as the body rates and
%   is in units of radians per second

%
% RETURN ARGUMENTS:
% pos_double_dot
% > This is a vector of length 3, and is computed using the equation of
%   motion for transaltion, it has units of meters per second squared
%
% psi_double_dot
% > This is a vector of length 3, and is computed using the equation of
%   motion for euler angle rotations, it has units of radians per second
%   squared
%
% w_dot
% > This is a vector of length 3, and is compute using the equation of
%   motion for body frame rotations, it has units of radians per second
%
%
% DATA FORMAT ASSUMPTIONS:
% > That the "p" is ordered as:
%   pos = [ x ; y ; z ];
% > And equivalently that the "psi_dot" is ordered as:
%   pos_dot = [ x_dot ; y_dot ; z_dot ];
% > That the "psi" is ordered as:
%   psi = [ roll ; pitch ; yaw ];
% > And equivalently that the "psi_dot" is ordered as:
%   psi_dot = [ roll_dot ; pitch_dot ; yaw_dot ];
% > That the "w" is ordered as:
%   w = [ w_x ; w_y ; w_z ];
%
% ----------------------------------------------------------------------- %

% Extract each euler angles
roll   =  psi(1);  % Roll
pitch  =  psi(2);  % Pitch
yaw    =  psi(3);  % Yaw

% Extract each euler anglular rates
roll_dot   =  psi_dot(1);  % Roll  angular velocity
pitch_dot  =  psi_dot(2);  % Pitch angular velocity
%yaw_dot    =  psi_dot(3); % Yaw   angular velocity, not needed


% Compute the rotation matrix from body frame to inertial frame:
R_B2I = [...
         cos(yaw)*cos(pitch)  ,  cos(yaw)*sin(pitch)*sin(roll)-sin(yaw)*cos(roll)  ,  cos(yaw)*sin(pitch)*cos(roll)+sin(yaw)*sin(roll)  ;...
         sin(yaw)*cos(pitch)  ,  sin(yaw)*sin(pitch)*sin(roll)+cos(yaw)*cos(roll)  ,  sin(yaw)*sin(pitch)*cos(roll)-cos(yaw)*sin(roll)  ;...
        -sin(pitch)         ,  cos(pitch)*sin(roll)                       ,  cos(pitch)*cos(roll)                        ...
    ];

% Compute the T inverse matrix:
T_inv = [...
        1  ,  sin(roll)*tan(pitch)  ,   cos(roll)*tan(pitch)  ;...
        0  ,  cos(roll)         ,  -sin(roll)         ;...
        0  ,  sin(roll)*sec(pitch)  ,   cos(roll)*sec(pitch)   ...
    ];

% Compute the time derivative of the T matrix:
T_dot = [...
        0  ,   0            ,  -pitch_dot*cos(pitch)                            ;...
        0  ,  -roll_dot*sin(roll)  ,   roll_dot*cos(roll)*cos(pitch)-pitch_dot*sin(roll)*sin(pitch)  ;...
        0  ,  -roll_dot*cos(roll)  ,  -roll_dot*sin(roll)*cos(pitch)-pitch_dot*cos(roll)*sin(pitch)   ...
    ];



% Implement the equation of motion for translation
pos_double_dot = (1/m) .* ( R_B2I * [0;0;sum(thrusts(:))] ) + [0;0;-g];



% Implement the equation of motion for body frame rotations
w_dot = J_inv * ( [layout(2,:);-layout(1,:);layout(3,:)] * thrusts - cross( w , J*w ) );



% Implement the equation of motion for euler angle rotations
psi_double_dot = T_inv * ( w_dot - T_dot * psi_dot );

end

== matlab function exercise02_simulation_model_solution_partA_R2025b/N-rotor vehicle model/Equations of Motion (Variants)/Version 2 of equations of motion in one shot/The full equations of motion implemented with one function ==
  data: g input; full_state_dot output; m input; J input; J_inv input; layout input; thrusts input; full_state input; body_rates output; body_accel output
function [full_state_dot,body_rates,body_accel] = fcn_eom(g,m,J,J_inv,layout,thrusts,full_state)
%
% ----------------------------------------------------------------------- %
% DESCRIPTION:
% This function implements the full equation of motion in one function to
% simplify the exposition.
%
%
% INPUT ARGUMENTS:
% m
% > This is the mass of the vehicle, in units of kilograms
%
% g
% > This is the acceleration due to gravity (typically 9.81), in units of
%   meters per second squared
%
% J
% > This is the moment of inertia matrix of the vehicle (it should be a
%   3-by3 matrix), the units of each element is kilogram meters squared
%
% J_inv
% > This is the inverse of the momement of inertia matrix, it is not
%   compute in this script to reduce the simulation run time slightly
%
% layout
% > This is a matrix that specifies the layout via the following format:
% nrotor_vehicle_layout = [...
%       x_1  ,  x_2  ,  ...  ,  x_{N-1}  ,  x_{N}  ;...
%       y_1  ,  y_2  ,  ...  ,  y_{N-1}  ,  y_{N}  ;...
%       c_1  ,  c_2  ,  ...  ,  c_{N-1}  ,  c_{N}   ...
%   ];
% where:
%   > x_i   is the x coordinate of propeller "i" relative to the CoG
%   > y_i   is the y coordinate of propeller "i" relative to the CoG
%   > c_i   is the thurst to torque coefficient of the propeller, with the
%           sign used to indicate the propeller's direction of rotation,
%           +ve indicates clock-wise propeller rotation.
%
% thrusts
% > This is a colulmn vector with length equal to the number of propellers
%   on the N-rotor vehicle, and each element represents the thrust force in
%   Newtons being produced by the respective propeller
%
% full_state
% > This is a vector of length 12 and is order as:
%   full_state[1:3]     the x,y,z posiiton of the body frame origin
%                       expressed in inertial frame coordinates, in units
%                       of [meters].
%
%   full_state[4:6]     the x,y,z linear velocity of the body frame origin
%                       expressed in inertial frame coordinates, in units
%                       of [meters per second].
%
%   full_state[7:9]     the roll, pitch, and yaw intrinsic Euler angles
%                       respectively, in units of [radians].
%
%   full_state[10:12]   the angular velocity of the roll, pitch, and yaw
%                       intrinsic Euler angles respectively, in units of
%                       [radians per second].
%
%
% RETURN ARGUMENTS:
% full_state_dot
% > This is a vector of length 12 and is ordered as:
%   full_state_dot[1:3]
%      - This is position dot and is taken directly as full_state[4:6]
%
%   full_state_dot[4:6]
%      - This is the position double dot and is computed using the equation
%        of motion for transaltion, it has units of [meters per second
%        squared]
%
%   full_state_dot[7:9]
%      - This is the angular velocity of the intrinsic Euler angles and is
%        taken directly as full_state[10:12]
%
%   full_state_dot[10:12]
%      - This is the angular accelerations of the intrinsic Euler angles
%        and is computed using the equation of motion for Euler angle
%        rotations, it has units of [radians per second squared]
%
% body_rates
% > This is a vector of length 3, each element represents the angular
%   velocity of the body frame as measured about the body frame's
%   coordinate axes, ordered as:
%   body_rates = [ w_x ; w_y ; w_z ];
%   In other words, this is exactly what is measured by a typical
%   strap-down Inertial Measurement Unit (IMU) that is attached to the body
%   of most all flying vehicles. It is computed directly from the "psi_dot"
%   by that is extracted from the "full_state" by applying the
%   transformation matrix "T". It has units of [radians per second];
%
% body_accel
% > This is a vector of length 3, each element represents the linear
%   accelerations of the body frame as measured along the body frame's
%   coordinate axes, i.e., this is exctly what is measured by a typical
%   strap-down Inertial Measurement Unit (IMU). It is computed directly
%   from the "pos_double_dot" by applying the rotation matrix from inertial
%   to body frame. It has units of [meters per second squared].
%
% ----------------------------------------------------------------------- %


% Extract the components of the full state
%pos      =  full_state(1:3);
pos_dot  =  full_state(4:6);
psi      =  full_state(7:9);
psi_dot  =  full_state(10:12);


% Extract each Euler angles
roll   =  psi(1);  % Roll  (gamma is the symbol used in the script)
pitch  =  psi(2);  % Pitch (beta  is the symbol used in the script)
yaw    =  psi(3);  % Yaw   (alpha is the symbol used in the script)


% Extract each Euler anglular rates
roll_dot   =  psi_dot(1);  % Roll  angular velocity
pitch_dot  =  psi_dot(2);  % Pitch angular velocity
%yaw_dot    =  psi_dot(3); % Yaw   angular velocity, not needed


% Compute the rotation matrix from body frame to inertial frame:
R_B2I = [...
            cos(yaw)*cos(pitch)  ,...
                cos(yaw)*sin(pitch)*sin(roll)-sin(yaw)*cos(roll)  ,...
                cos(yaw)*sin(pitch)*cos(roll)+sin(yaw)*sin(roll)   ...
            ;...
            sin(yaw)*cos(pitch)  ,...
                sin(yaw)*sin(pitch)*sin(roll)+cos(yaw)*cos(roll)  ,...
                sin(yaw)*sin(pitch)*cos(roll)-cos(yaw)*sin(roll)   ...
            ;...
            -sin(pitch)  ,...
                cos(pitch)*sin(roll)  ,...
                cos(pitch)*cos(roll)   ...
    ];


% Compute the T matrix:
T = [...
        1  ,  0          ,  -sin(pitch)            ;...
        0  ,  cos(roll)  ,   sin(roll)*cos(pitch)  ;...
        0  , -sin(roll)  ,   cos(roll)*cos(pitch)   ...
    ];


% Compute the T inverse matrix:
T_inv = [...
        1  ,  sin(roll)*tan(pitch)  ,   cos(roll)*tan(pitch)  ;...
        0  ,  cos(roll)             ,  -sin(roll)             ;...
        0  ,  sin(roll)*sec(pitch)  ,   cos(roll)*sec(pitch)   ...
    ];


% Compute the time derivative of the T matrix:
T_dot = [...
        0  ,   0                   ,  -pitch_dot*cos(pitch)                                          ;...
        0  ,  -roll_dot*sin(roll)  ,   roll_dot*cos(roll)*cos(pitch)-pitch_dot*sin(roll)*sin(pitch)  ;...
        0  ,  -roll_dot*cos(roll)  ,  -roll_dot*sin(roll)*cos(pitch)-pitch_dot*cos(roll)*sin(pitch)   ...
    ];


% Implement the equation of motion for translation
pos_double_dot = (1/m) .* ( R_B2I * [0;0;sum(thrusts(:))] ) + [0;0;-g];


% Compute the body rates from the Euler angluar rates
w = T * psi_dot;


% Implement the equation of motion for body frame rotations
w_dot = J_inv * ( [layout(2,:);-layout(1,:);layout(3,:)] * thrusts - cross( w , J*w ) );


% Implement the equation of motion for Euler angle rotations
psi_double_dot = T_inv * ( w_dot - T_dot * psi_dot );


% Put together the "full_state_dot" return variable
full_state_dot = [...
        pos_dot ;...
        pos_double_dot ;...
        psi_dot ;...
        psi_double_dot ...
    ];


% Put together the "body_rates" return variable
body_rates = w;


% Finally compute the accelerations in the body frame
% > by "simply" rotating the inertial frame linear accelerations, i.e.,
%   "pos_double_dot", from the inertial frame into the body frame
% > do you need to account for the fact that the body frame accelerations
%   are measured in a rotating frame?
body_accel = transpose(R_B2I) * psi_double_dot;


end
